simulink model "System"  (R2018b)
settings: Solver=VariableStepAuto  StartTime=0.0  StopTime=30.0  RelTol=1e-3
undefined symbols (not defined in the file or in its folder): Ts
libraries: mpclib x1, vrlib x1
settings Model: Creator=Yahya  LastModifiedBy=Yahya

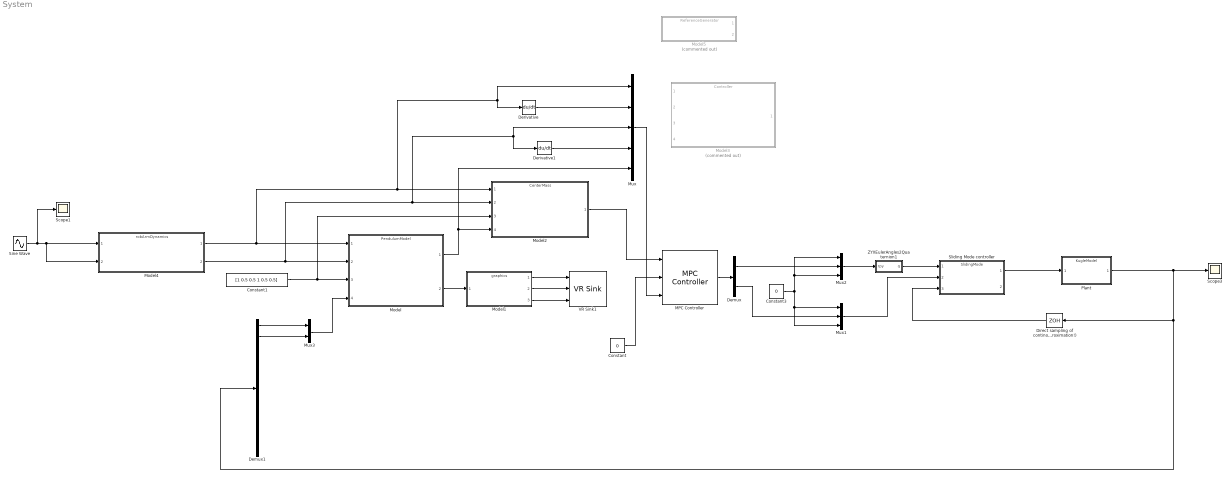
== system System ==
  Constant : Constant  Value=0
  Constant1 : Constant  Value=[1 0.5 0.5 1 0.5 0.5]
  Constant3 : Constant  Value=0
  Demux : Demux  Outputs=2
  Demux1 : Demux  Outputs=12
  Derivative : Derivative
  Derivative1 : Derivative
  Direct sampling of continous states (simple/approximation!) : ZeroOrderHold  SampleTime=Ts
  MPC Controller : mpclib/MPC Controller  SCDEnableBlockLinearizationSpecification=on  is_multiple=0  enable_value=0  return_u0=off  updateMPCinCallerWorkspace=on  md_inport=on  mv_inport=off  return_cost=off  return_mvseq=off  return_qpstatus=off  return_xseq=off  return_state=off  return_ovseq=off  state_inport=off  umin_inport=off  umax_inport=off  ymin_inport=off  ymax_inport=off  cc_inport=off  ywt_inport=off  uwt_inport=off  duwt_inport=off  rhoeps_inport=off  uref_inport=off  n_ts=0.01  n_p=50  n_mv=2  n_md=6  n_ud=0  n_mo=1  n_uo=0  BlockDataType=double  SampleTimeInherited=off  switch_inport=off
  Model : ModelReference  ModelNameDialog=PendulumModel.slx  SimulationMode=Normal  ModelReferenceVersion=1.20
  Model1 : ModelReference  ModelNameDialog=graphics.slx  SimulationMode=Normal  ModelReferenceVersion=1.7
  Model2 : ModelReference  ModelNameDialog=CenterMass.slx  SimulationMode=Normal  ModelReferenceVersion=1.9
  Model3 : ModelReference  Commented=on  ModelNameDialog=Controller.slx  SimulationMode=Normal  ModelReferenceVersion=1.9
  Model4 : ModelReference  ModelNameDialog=robArmDynamics.slx  SimulationMode=Normal  ModelReferenceVersion=1.3
  Model5 : ModelReference  Commented=on  ModelNameDialog=ReferenceGenerator  SimulationMode=Normal  ModelReferenceVersion=1.7
  Mux : Mux  Inputs=5
  Mux1 : Mux  Inputs=3
  Mux2 : Mux  Inputs=3
  Mux3 : Mux  Inputs=2
  Plant : ModelReference  ModelNameDialog=KugleModel  SimulationMode=Normal  ModelReferenceVersion=1.2093
  Scope1 : Scope
  Scope3 : Scope
  Sine Wave : Sin  Amplitude=pi/18  Frequency=pi/9  SampleTime=0
  Sliding Mode controller : ModelReference  ModelNameDialog=SlidingMode  SimulationMode=Normal  ModelReferenceVersion=1.48
  VR Sink1 : vrlib/VR Sink  InstantiateOnLoad=on  SampleTime=0.1  ViewEnable=on  RemoteChange=off  RemoteView=off  FieldsWritten=JOINT_1.rotation.4.1.1.double#JOINT_2.rotation.4.1.1.double#JOINT_3.rotation.4.1.1.double  WorldFileName=Pendel3D0.wrl  AutoView=off  VideoDimensions=[]  AllowVariableSize=off  FigureProperties="{'Position', 'Name', 'Viewpoint', 'CameraBound', 'CameraDirection', 'CameraPosition', 'CameraUpVector', 'ZoomFactor', 'Antialiasing', 'Headlight', 'Lighting', 'NavPanel', 'Sound', 'StatusBar', 'Stereo3D', 'Stereo3DCameraOffset', 'Stereo3DHIT', 'ToolBar', 'Textures', 'Transparency', 'Triad', 'Wireframe', 'NavZones', 'NavMode', 'NavSpeed', 'CaptureFileFormat', 'CaptureFileName', 'Record2DCompressMethod', 'Record2DCompressQuality', 'Record2D', 'Record2DFileName', 'Record2DFPS'; [5.0000000000000000e+00   9.2000000000000000e+01   5.7600000000000000e+02   3.5000000000000000e+02], '', '', 'on', [0.0000000000000000e+00   0.0000000000000000e+00  -1.0000000000000000e+00], [0.0000000000000000e+00   0.0000000000000000e+00   1.0000000000000000e+01], [0.0000000000000000e+00   1.0000000000000000e+00   0.0000000000000000e+00], [1.0000000000000000e+00], 'on', 'on', 'on', 'halfbar', 'on', 'on', 'off', [1.0000000149011612e-01], [0.0000000000000000e+00], 'on', 'on', 'on', 'none', 'off', 'off', 'fly', 'normal', 'tif', '%f_anim_%n.tif', 'auto', [7.5000000000000000e+01], 'off', '%f_anim_%n.avi', 'auto'}"
      settings: SourceProductBaseCode=VR
  ZYXEulerAngles2Quaternion1 : MATLAB Function  TreatAsAtomicUnit=on
  wires:
  Model4/2 -> Mux/3, Derivative1/1, Model2/2, Model/2
  Model/1 -> Mux/5, Model2/4
  Constant1/1 -> Model/3, Model2/3
  Model2/1 -> MPC Controller/1
  Model1/1 -> VR Sink1/1
  Model1/2 -> VR Sink1/2
  Model1/3 -> VR Sink1/3
  Model/2 -> Model1/1
  Sine Wave/1 -> Scope1/1, Model4/2, Model4/1
  Direct sampling of continous states (simple/approximation!)/1 -> Sliding Mode controller/3
  Sliding Mode controller/1 -> Plant/1
  Plant/1 -> Demux1/1, Direct sampling of continous states (simple/approximation!)/1, Scope3/1
  Mux1/1 -> Sliding Mode controller/2
  ZYXEulerAngles2Quaternion1/1(q) -> Sliding Mode controller/1
  Mux2/1 -> ZYXEulerAngles2Quaternion1/1(rpy)
  Constant3/1 -> Mux2/1, Mux2/3, Mux1/3, Mux1/1
  Derivative/1 -> Mux/2
  Model4/1 -> Mux/1, Derivative/1, Model2/1, Model/1
  Derivative1/1 -> Mux/4
  MPC Controller/1 -> Demux/1
  Demux/1 -> Mux2/2
  Demux/2 -> Mux1/2
  Mux/1 -> MPC Controller/3
  Mux3/1 -> Model/4
  Demux1/1 -> Mux3/1
  Demux1/2 -> Mux3/2
  Constant/1 -> MPC Controller/2

== matlab function System/ZYXEulerAngles2Quaternion1 ==
  data: rpy input size=3; q output size=4
function q = ZYXEulerAngles2Quaternion(rpy)
    q = ZYXEulerAngles2Quaternion(rpy);
end
